simulink model "P6"  (R2024a)
settings: Solver=ode45  StartTime=0.0  StopTime=5  RelTol=1e-3
settings Model: Creator=ahmad  LastModifiedBy=ahmad

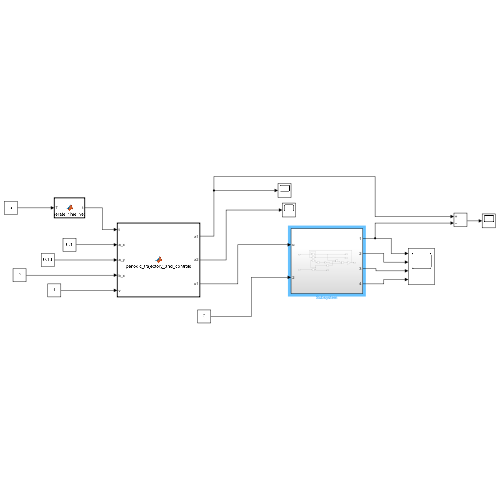
[thumbnail: Simulink's stored preview of the top-level diagram]
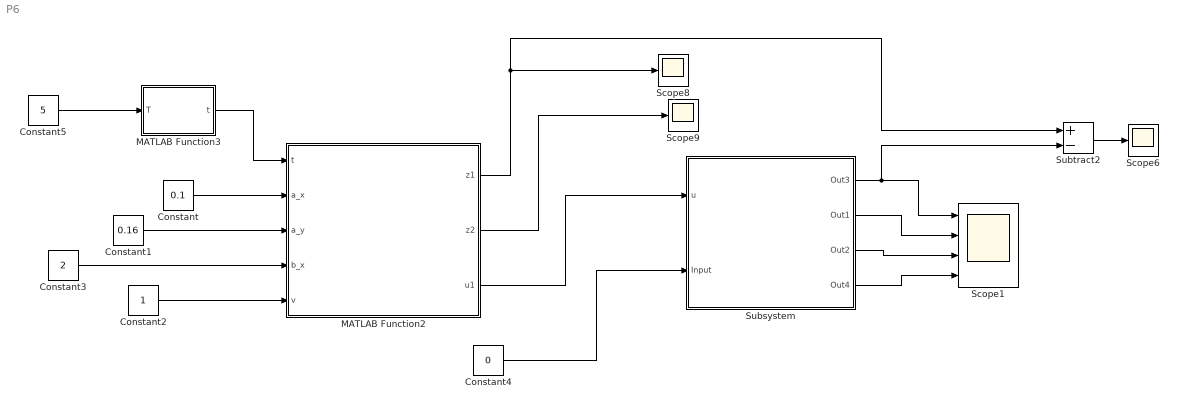
== system P6 ==
  Constant : Constant  Value=0.1
  Constant1 : Constant  Value=0.16
  Constant2 : Constant
  Constant3 : Constant  Value=2
  Constant4 : Constant  Value=0
  Constant5 : Constant  Value=5
  MATLAB Function2 : MATLAB Function  TreatAsAtomicUnit=on
  MATLAB Function3 : MATLAB Function  TreatAsAtomicUnit=on
  Scope1 : Scope  NumInputPorts=4
  Scope6 : Scope
  Scope8 : Scope
  Scope9 : Scope
  Subsystem : Subsystem
  Subtract2 : Sum  Inputs=+-
  wires:
  Subtract2/1 -> Scope6/1
  Constant5/1 -> MATLAB Function3/1(T)
  MATLAB Function3/1(t) -> MATLAB Function2/1(t)
  Constant/1 -> MATLAB Function2/2(a_x)
  Constant1/1 -> MATLAB Function2/3(a_y)
  Constant2/1 -> MATLAB Function2/5(v)
  Constant3/1 -> MATLAB Function2/4(b_x)
  MATLAB Function2/1(z1) -> Subtract2/1, Scope8/1
  MATLAB Function2/2(z2) -> Scope9/1
  MATLAB Function2/3(u1) -> Subsystem/1(u)
  Constant4/1 -> Subsystem/2(Input)
  Subsystem/1(Out3) -> Subtract2/2, Scope1/1
  Subsystem/2(Out1) -> Scope1/2
  Subsystem/3(Out2) -> Scope1/3
  Subsystem/4(Out4) -> Scope1/4

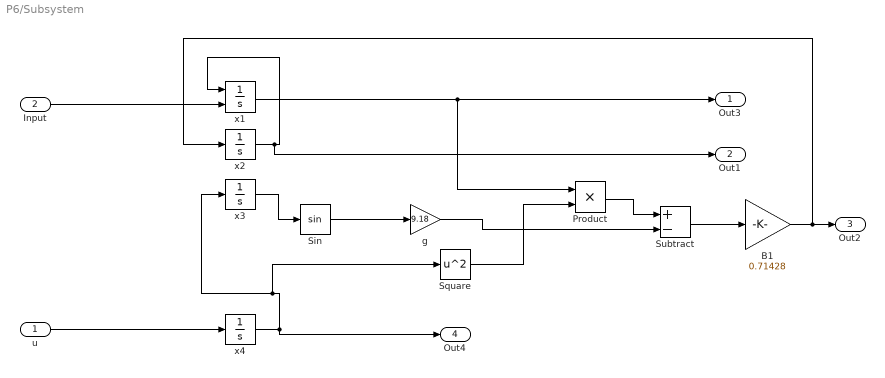
== system P6/Subsystem ==
  u : Inport
  Input : Inport  Port=2
  B1 : Gain  Gain=0.71428
  Product : Product
  Sin : Trigonometry
  Square : Math  Operator=square
  Subtract : Sum  Inputs=+-
  g : Gain  Gain=9.18
  x1 : Integrator  InitialConditionSource=external
  x2 : Integrator
  x3 : Integrator
  x4 : Integrator
  Out3 : Outport
  Out1 : Outport  Port=2
  Out2 : Outport  Port=3
  Out4 : Outport  Port=4
  wires:
  x2/1 -> Out1/1, x1/1
  x4/1 -> Square/1, x3/1, Out4/1
  x1/1 -> Product/1, Out3/1
  u/1 -> x4/1
  Input/1 -> x1/2
  Square/1 -> Product/2
  x3/1 -> Sin/1
  Product/1 -> Subtract/1
  Sin/1 -> g/1
  g/1 -> Subtract/2
  Subtract/1 -> B1/1
  B1/1 -> x2/1, Out2/1

== matlab function P6/MATLAB Function2 ==
  data: t input; z1 output; a_x input; a_y input; b_x input; v input; z2 output; u1 output
function [z1, z2, u1] = periodic_trajectory_and_controls(t, a_x, a_y, b_x, v)
% PERIODIC_TRAJECTORY_AND_CONTROLS Computes periodic desired trajectories and controls
% for the ball-on-plate system for both x- and y-directions.
%
% Inputs:
%   t     - Time variable (scalar or vector)
%   a_x   - Amplitude in x-direction
%   a_y   - Amplitude in y-direction
%   b_x   - Parameter defining the trajectory type (1 = circle, 2 = eight, 4 = double eight)
%   v     - Angular velocity (rad/s)
%
% Outputs:
%   z1    - Desired trajectory for x-direction
%   z2    - Desired trajectory for y-direction
%   u1    - Control input for x-direction (fourth derivative of z1)
%   u2    - Control input for y-direction (fourth derivative of z2)

    % Desired trajectory in x-direction (z1)
    z1 = a_x * sin(b_x * v * t);
    % Desired trajectory in y-direction (z2)
    z2 = a_y * cos(v * t);

    % First derivatives
    dz1 = a_x * b_x * v * cos(b_x * v * t);
    dz2 = -a_y * v * sin(v * t);

    % Second derivatives
    ddz1 = -a_x * b_x^2 * v^2 * sin(b_x * v * t);
    ddz2 = -a_y * v^2 * cos(v * t);

    % Third derivatives
    dddz1 = -a_x * b_x^3 * v^3 * cos(b_x * v * t);
    dddz2 = a_y * v^3 * sin(v * t);

    % Fourth derivatives (controls)
    u1 = a_x * b_x^4 * v^4 * sin(b_x * v * t);
    u2 = a_y * v^4 * cos(v * t);

end

== matlab function P6/MATLAB Function3 ==
  data: T input; t output
function t = generate_time_vector(T)
    % Inputs: T is the total time
    % Outputs: t is a time vector
    t = linspace(0, T, 100);
end
